simulink model "quad_control_elev8_sAttit"  (Simulink 8.7)
settings: Solver=VariableStepAuto  StartTime=0.0  StopTime=200  FixedStep=0.01  MaxStep=0.1  RelTol=1e-3
InitFcn:
  | ganho=50;
  | z1=0.005;
  | z2=0.001;
  | P_X = (z1+z2)*ganho;      I_X = z1*z2*ganho;     D_X  = ganho;
  | P_Y = (z1+z2)*ganho;      I_Y = z1*z2*ganho;      D_Y  = ganho;
  | P_Z = 32;       I_Z = 3;          D_Z = 15;
  | % --------------------------
  | 
  | global clientID;
  | clientID=-1;
undefined symbols (not defined in the file or in its folder): Angular, Linear, sigbuilder_block
libraries: dspsigops x7, robotlib x7, simulink_extras x3, aerolibutil x1, aerolibtransform2 x1
settings Model: Creator=kleber  LastModifiedBy=kleber
settings DataIOCC: LimitDataPoints=off
settings DebuggingCC: UnderspecifiedInitializationDetection=Simplified  MergeDetectMultiDrivingBlocksExec=error  SolverPrmCheckMsg=warning
settings ConfigComp: CovSFcnEnable=off

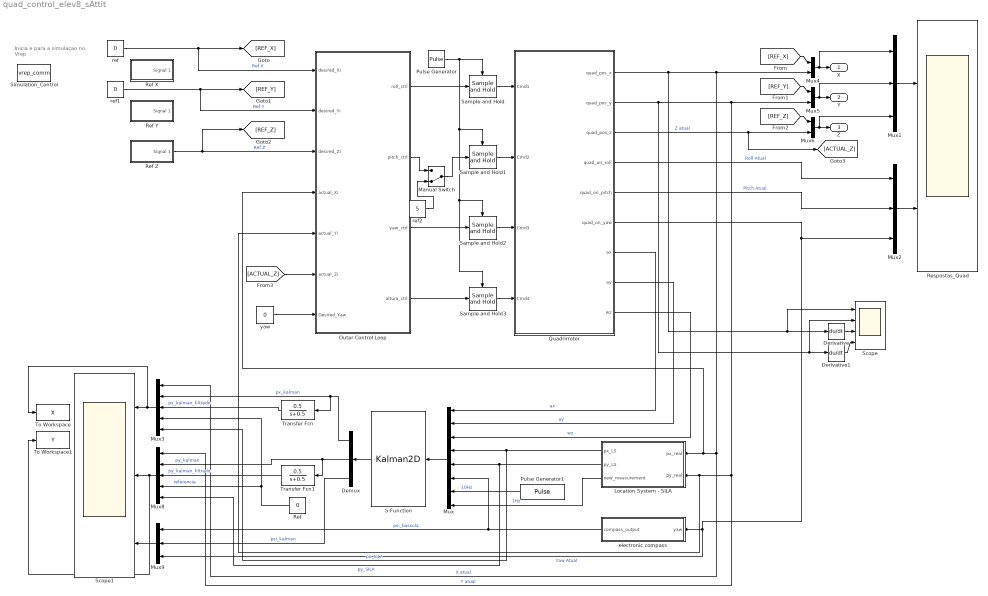
== system quad_control_elev8_sAttit ==
  note: Inicia e para a simulaçao no Vrep
  Demux : Demux  Outputs=3
  Derivative : Derivative
  Derivative1 : Derivative
  Location System - SILA : Subsystem
  Manual Switch : ManualSwitch  CurrentSetting=0
  Mux : Mux  Inputs=8
  Mux1 : Mux  Inputs=3
  Mux2 : Mux  Inputs=3
  Mux3 : Mux  Inputs=5
  Mux4 : Mux  Inputs=2
  Mux5 : Mux  Inputs=2
  Mux6 : Mux  Inputs=2
  Mux8 : Mux  Inputs=5
  Mux9 : Mux  Inputs=3
  Outer Control Loop : Subsystem
  Pulse Generator : DiscretePulseGenerator  PulseType=Time based  Period=0.1  PulseWidth=20  PhaseDelay=0.02
  Pulse Generator1 : DiscretePulseGenerator  PulseType=Time based  Period=0.1  PulseWidth=20
  Quadrirrotor : Subsystem
  Ref : Constant  Value=0
  Ref X : Subsystem  Tag=STV Subsys  LoadFcn=sigbuilder_block('load');  StartFcn=sigbuilder_block('start');  StopFcn=sigbuilder_block('stop');  ClipboardFcn=sigbuilder_block('clipboard');  mask(Sigbuilder block){}
      mask help: Sigbuilder GUI
      mask init:
      | if ~strcmp(get_param(bdroot(gcbh),'SimulationStatus'),'stopped') tuvar = sigbuilder_block('maskInit'); end
      settings: CopyFcn=sigbuilder_block('copy');  DeleteFcn=sigbuilder_block('delete');  ModelCloseFcn=sigbuilder_block('modelClose');  PreSaveFcn=sigbuilder_block('preSave');  PauseFcn=sigbuilder_block('pause')  ContinueFcn=sigbuilder_block('continue')  NameChangeFcn=sigbuilder_block('namechange');  OpenFcn=sigbuilder_block('open',[1024.5 -192 960 708.75 ]);  CloseFcn=sigbuilder_block('close');
      mask Display: plot(0,0,100,100,[10,10,40,40,10],[80,20,20,80,80],[40,10],[50,50], [40,27,10],[65,72,56],[40,25,25,10],[28,28,43,43]);
  Ref Y : Subsystem  Tag=STV Subsys  LoadFcn=sigbuilder_block('load');  StartFcn=sigbuilder_block('start');  StopFcn=sigbuilder_block('stop');  ClipboardFcn=sigbuilder_block('clipboard');  mask(Sigbuilder block){}
      mask help: Sigbuilder GUI
      mask init:
      | if ~strcmp(get_param(bdroot(gcbh),'SimulationStatus'),'stopped') tuvar = sigbuilder_block('maskInit'); end
      settings: CopyFcn=sigbuilder_block('copy');  DeleteFcn=sigbuilder_block('delete');  ModelCloseFcn=sigbuilder_block('modelClose');  PreSaveFcn=sigbuilder_block('preSave');  PauseFcn=sigbuilder_block('pause')  ContinueFcn=sigbuilder_block('continue')  NameChangeFcn=sigbuilder_block('namechange');  OpenFcn=sigbuilder_block('open',[39.75 0 984.75 516.75 ]);  CloseFcn=sigbuilder_block('close');
      mask Display: plot(0,0,100,100,[10,10,40,40,10],[80,20,20,80,80],[40,10],[50,50], [40,27,10],[65,72,56],[40,25,25,10],[28,28,43,43]);
  Ref Z : Subsystem  Tag=STV Subsys  LoadFcn=sigbuilder_block('load');  StartFcn=sigbuilder_block('start');  StopFcn=sigbuilder_block('stop');  ClipboardFcn=sigbuilder_block('clipboard');  mask(Sigbuilder block){}
      mask help: Sigbuilder GUI
      mask init:
      | if ~strcmp(get_param(bdroot(gcbh),'SimulationStatus'),'stopped') tuvar = sigbuilder_block('maskInit'); end
      settings: CopyFcn=sigbuilder_block('copy');  DeleteFcn=sigbuilder_block('delete');  ModelCloseFcn=sigbuilder_block('modelClose');  PreSaveFcn=sigbuilder_block('preSave');  PauseFcn=sigbuilder_block('pause')  ContinueFcn=sigbuilder_block('continue')  NameChangeFcn=sigbuilder_block('namechange');  OpenFcn=sigbuilder_block('open',[43.5 0 981 277.5 ]);  CloseFcn=sigbuilder_block('close');
      mask Display: plot(0,0,100,100,[10,10,40,40,10],[80,20,20,80,80],[40,10],[50,50], [40,27,10],[65,72,56],[40,25,25,10],[28,28,43,43]);
  Respostas_Quad : Scope  NumInputPorts=2
  S-Function : S-Function  FunctionName=Kalman2D  SFunctionDeploymentMode=off  EnableBusSupport=off
  Sample and Hold{,1..3} (4 alike) : dspsigops/Sample and Hold  trig=Rising edge  initCond=0  latchinput=off
  Scope : Scope  NumInputPorts=4
  Scope1 : Scope  NumInputPorts=3
  Simulation_Control : S-Function  FunctionName=vrep_comm  SFunctionDeploymentMode=off  EnableBusSupport=off
  To Workspace : ToWorkspace  VariableName=X  SaveFormat=Timeseries  SampleTime=-1
  To Workspace1 : ToWorkspace  VariableName=Y  SaveFormat=Timeseries  SampleTime=-1
  Transfer Fcn : TransferFcn  Numerator=[0.5]  Denominator=[1 0.5]
  Transfer Fcn1 : TransferFcn  Numerator=[0.5]  Denominator=[1 0.5]
  electronic compass : Subsystem
  ref : Constant  Value=0
  ref1 : Constant  Value=0
  ref2 : Constant  Value=5
  yaw : Constant  Value=0
  X : Outport
  Y : Outport  Port=2
  Z : Outport  Port=3
  wires:
  Mux1/1 -> Respostas_Quad/1
  Mux2/1 -> Respostas_Quad/2
  Quadrirrotor/5(quad_ori_pitch) -> Mux2/2  "Pitch Atual"
  Quadrirrotor/4(quad_ori_roll) -> Mux2/1  "Roll Atual"
  Quadrirrotor/3(quad_pos_z) -> Mux6/2, [ACTUAL_Z]  "Z atual"
  Quadrirrotor/6(quad_ori_yaw) -> Mux9/3, electronic compass/1(yaw), Mux2/3  "Yaw Atual"
  Pulse Generator/1 -> Sample and Hold2/Trigger, Sample and Hold3/Trigger, Sample and Hold1/Trigger, Sample and Hold/Trigger
  Outer Control Loop/4(altura_ctrl) -> Sample and Hold3/1
  Mux4/1 -> X/1, Mux1/1
  Mux5/1 -> Mux1/2, Y/1
  Mux6/1 -> Mux1/3, Z/1
  Outer Control Loop/3(yaw_ctrl) -> Sample and Hold2/1
  Manual Switch/1 -> Sample and Hold1/1
  Outer Control Loop/1(roll_ctrl) -> Sample and Hold/1
  yaw/1 -> Outer Control Loop/7(Desired_Yaw)
  Sample and Hold3/1 -> Quadrirrotor/4(Cmd4)
  Ref Z/1(Signal 1) -> [REF_Z], Outer Control Loop/3(desired_Zi)  "Ref Z"
  Sample and Hold2/1 -> Quadrirrotor/3(Cmd3)
  Mux/1 -> S-Function/1
  Quadrirrotor/7(ax) -> Mux/1  "ax"
  Quadrirrotor/8(ay) -> Mux/2  "ay"
  Quadrirrotor/9(wz) -> Mux/3  "wz"
  Location System - SILA/1(px_LS) -> Mux/4, Mux3/5  "px_SILA"
  Location System - SILA/2(py_LS) -> Mux8/5, Mux/5  "py_SILA"
  [REF_X] -> Mux4/1
  [REF_Y] -> Mux5/1
  [REF_Z] -> Mux6/1
  [ACTUAL_Z] -> Outer Control Loop/6(actual_Zi)
  electronic compass/1(compass_output) -> Mux/6, Mux9/1  "psi_bussola"
  Location System - SILA/3(new_measurement) -> Mux/8  "1Hz"
  S-Function/1 -> Demux/1
  Quadrirrotor/2(quad_pos_y) -> Scope/2, Derivative1/1, Mux5/2, Outer Control Loop/5(actual_Yi), Location System - SILA/2(py_real), Mux8/1  "Y atual"
  Quadrirrotor/1(quad_pos_x) -> Scope/1, Derivative/1, Mux4/2, Outer Control Loop/4(actual_Xi), Location System - SILA/1(px_real), Mux3/1  "X atual"
  Demux/1 -> Transfer Fcn/1, Mux3/2  "px_kalman"
  Mux8/1 -> To Workspace1/1, Scope1/2
  Demux/2 -> Transfer Fcn1/1, Mux8/2  "py_kalman"
  Mux9/1 -> Scope1/3
  Demux/3 -> Mux9/2  "psi_kalman"
  Sample and Hold/1 -> Quadrirrotor/1(Cmd1)
  Transfer Fcn1/1 -> Mux8/3  "py_kalman_filtrado"
  Transfer Fcn/1 -> Mux3/3  "px_kalman_filtrado"
  Sample and Hold1/1 -> Quadrirrotor/2(Cmd2)
  Ref/1 -> Mux3/4, Mux8/4  "referencia"
  Pulse Generator1/1 -> Mux/7  "10Hz"
  ref/1 -> Outer Control Loop/1(desired_Xi), [REF_X]  "Ref X"
  ref1/1 -> Outer Control Loop/2(desired_Yi), [REF_Y]  "Ref Y"
  Mux3/1 -> To Workspace/1, Scope1/1
  Outer Control Loop/2(pitch_ctrl) -> Manual Switch/1
  ref2/1 -> Manual Switch/2
  Derivative/1 -> Scope/3
  Derivative1/1 -> Scope/4

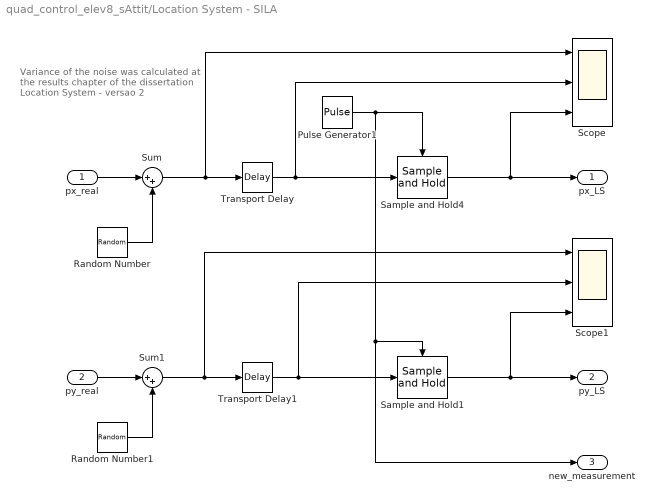
== system quad_control_elev8_sAttit/Location System - SILA ==
  note: Variance of the noise was calculated
      | at the results chapter of the dissertation
      | Location System - versao 2
  px_real : Inport
  py_real : Inport  Port=2
  Pulse Generator1 : DiscretePulseGenerator  PulseType=Time based  Period=1  PulseWidth=10
  Random Number : RandomNumber  Variance=0.0010  SampleTime=1
  Random Number1 : RandomNumber  Variance=0.0012  SampleTime=1
  Sample and Hold1 : dspsigops/Sample and Hold  trig=Rising edge  initCond=0  latchinput=off
  Sample and Hold4 : dspsigops/Sample and Hold  trig=Rising edge  initCond=0  latchinput=off
  Scope : Scope  NumInputPorts=3
  Scope1 : Scope  NumInputPorts=3
  Sum : Sum  Inputs=|++
  Sum1 : Sum  Inputs=|++
  Transport Delay : TransportDelay  DelayTime=0.5
  Transport Delay1 : TransportDelay  DelayTime=0.5
  px_LS : Outport
  py_LS : Outport  Port=2
  new_measurement : Outport  Port=3
  wires:
  Sample and Hold4/1 -> px_LS/1, Scope/3
  Sum/1 -> Transport Delay/1, Scope/1
  Transport Delay/1 -> Sample and Hold4/1, Scope/2
  Sample and Hold1/1 -> py_LS/1, Scope1/3
  Transport Delay1/1 -> Sample and Hold1/1, Scope1/2
  Pulse Generator1/1 -> Sample and Hold4/Trigger, new_measurement/1, Sample and Hold1/Trigger
  px_real/1 -> Sum/1
  Sum1/1 -> Scope1/1, Transport Delay1/1
  py_real/1 -> Sum1/1
  Random Number1/1 -> Sum1/2
  Random Number/1 -> Sum/2

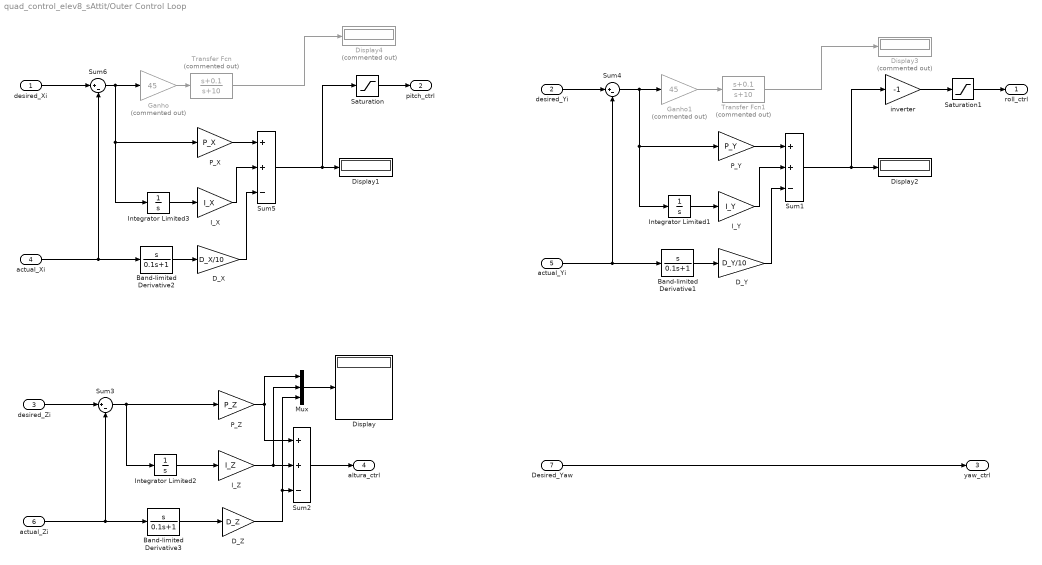
== system quad_control_elev8_sAttit/Outer Control Loop ==
  desired_Xi : Inport
  desired_Yi : Inport  Port=2
  desired_Zi : Inport  Port=3
  actual_Xi : Inport  Port=4
  actual_Yi : Inport  Port=5
  actual_Zi : Inport  Port=6
  Desired_Yaw : Inport  Port=7
  Band-limited Derivative1 : TransferFcn  Numerator=[1 0]  Denominator=[0.1 1]
  Band-limited Derivative2 : TransferFcn  Numerator=[1 0]  Denominator=[0.1 1]
  Band-limited Derivative3 : TransferFcn  Numerator=[1 0]  Denominator=[0.1 1]
  D_X : Gain  Gain=D_X/10
  D_Y : Gain  Gain=D_Y/10
  D_Z : Gain  Gain=D_Z
  Display : Display
  Display1 : Display
  Display2 : Display
  Display3 : Display  Commented=on
  Display4 : Display  Commented=on
  Ganho : Gain  Commented=on  Gain=45
  Ganho1 : Gain  Commented=on  Gain=45
  I_X : Gain  Gain=I_X
  I_Y : Gain  Gain=I_Y
  I_Z : Gain  Gain=I_Z
  Integrator Limited1 : Integrator  LimitOutput=on  UpperSaturationLimit=0.5  LowerSaturationLimit=-0.5
  Integrator Limited2 : Integrator  InitialCondition=1  LimitOutput=on  UpperSaturationLimit=10  LowerSaturationLimit=0
  Integrator Limited3 : Integrator  LimitOutput=on  UpperSaturationLimit=0.5  LowerSaturationLimit=-0.5
  Mux : Mux  Inputs=3
  P_X : Gain  Gain=P_X
  P_Y : Gain  Gain=P_Y
  P_Z : Gain  Gain=P_Z
  Saturation : Saturate  UpperLimit=2  LowerLimit=-2
  Saturation1 : Saturate  UpperLimit=2  LowerLimit=-2
  Sum1 : Sum  Inputs=++-
  Sum2 : Sum  Inputs=++-
  Sum3 : Sum  Inputs=|+-
  Sum4 : Sum  Inputs=|+-
  Sum5 : Sum  Inputs=++-
  Sum6 : Sum  Inputs=|+-
  Transfer Fcn : TransferFcn  Commented=on  Numerator=[1 0.1]  Denominator=[1 10]
  Transfer Fcn1 : TransferFcn  Commented=on  Numerator=[1 0.1]  Denominator=[1 10]
  inverter : Gain  Gain=-1
  roll_ctrl : Outport
  pitch_ctrl : Outport  Port=2
  yaw_ctrl : Outport  Port=3
  altura_ctrl : Outport  Port=4
  wires:
  Sum2/1 -> altura_ctrl/1
  Desired_Yaw/1 -> yaw_ctrl/1
  Saturation/1 -> pitch_ctrl/1
  inverter/1 -> Saturation1/1
  Saturation1/1 -> roll_ctrl/1
  Mux/1 -> Display/1
  Sum3/1 -> Integrator Limited2/1, P_Z/1
  P_Z/1 -> Sum2/1, Mux/1
  D_Z/1 -> Mux/3, Sum2/3
  Band-limited Derivative3/1 -> D_Z/1
  I_Z/1 -> Mux/2, Sum2/2
  Integrator Limited3/1 -> I_X/1
  P_X/1 -> Sum5/1
  D_X/1 -> Sum5/3
  actual_Xi/1 -> Band-limited Derivative2/1, Sum6/2
  desired_Xi/1 -> Sum6/1
  I_X/1 -> Sum5/2
  Integrator Limited2/1 -> I_Z/1
  Integrator Limited1/1 -> I_Y/1
  P_Y/1 -> Sum1/1
  D_Y/1 -> Sum1/3
  actual_Yi/1 -> Band-limited Derivative1/1, Sum4/2
  desired_Yi/1 -> Sum4/1
  I_Y/1 -> Sum1/2
  actual_Zi/1 -> Band-limited Derivative3/1, Sum3/2
  desired_Zi/1 -> Sum3/1
  Sum5/1 -> Saturation/1, Display1/1
  Sum6/1 -> Integrator Limited3/1, P_X/1, Ganho/1
  Ganho/1 -> Transfer Fcn/1
  Ganho1/1 -> Transfer Fcn1/1
  Sum4/1 -> Integrator Limited1/1, P_Y/1, Ganho1/1
  Sum1/1 -> inverter/1, Display2/1
  Band-limited Derivative2/1 -> D_X/1
  Band-limited Derivative1/1 -> D_Y/1
  Transfer Fcn/1 -> Display4/1
  Transfer Fcn1/1 -> Display3/1

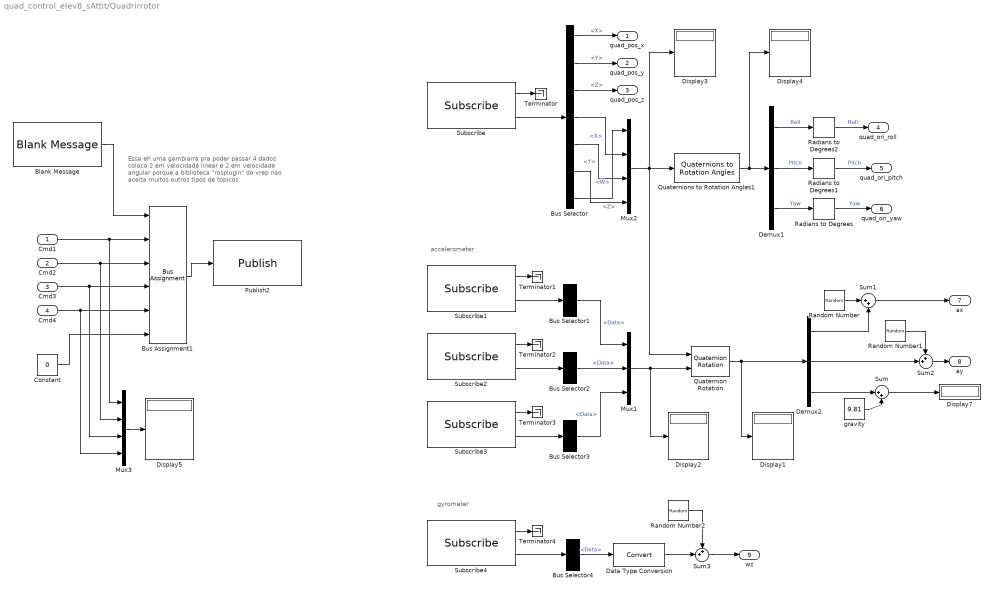
== system quad_control_elev8_sAttit/Quadrirrotor ==
  note: accelerometer
  note: Essa eh uma gambiarra pra poder passar 4 dados coloco 2 em velocidade linear e 2 em velocidade angular porque a biblioteca "rosplugin" do vrep nao aceita muitos outros tipos de topicos
  note: gyrometer
  Cmd1 : Inport
  Cmd2 : Inport  Port=2
  Cmd3 : Inport  Port=3
  Cmd4 : Inport  Port=4
  Blank Message : robotlib/Blank Message  SourceLibraryInfo=This block requires Robotics System Toolbox  messageType=geometry_msgs/Twist  SampleTime=inf
  Bus Assignment1 : BusAssignment  DialogController=Simulink.DDGSource_BusAssignment  AssignedSignals=Linear.X,Linear.Y,Angular.X,Angular.Y,Angular.Z
  Bus Selector : BusSelector  OutputSignals=Pose.Position.X,Pose.Position.Y,Pose.Position.Z,Pose.Orientation.X,Pose.Orientation.Y,Pose.Orientation.Z,Pose.Orientation.W
  Bus Selector{1..4} (4 alike) : BusSelector  OutputSignals=Data
  Constant : Constant  Value=0
  Data Type Conversion : DataTypeConversion
  Demux1 : Demux  Outputs=3
  Demux2 : Demux  Outputs=3
  Display{1..5,7} (6 alike) : Display
  Mux1 : Mux  Inputs=3
  Mux2 : Mux
  Mux3 : Mux
  Publish2 : robotlib/Publish  SourceLibraryInfo=This block requires Robotics System Toolbox  topicSource=Select from ROS network  topic=/control_signals  messageType=geometry_msgs/Twist  messageQueueLength=105
  Quaternion Rotation : aerolibutil/Quaternion Rotation
  Quaternions to Rotation Angles1 : aerolibtransform2/Quaternions to Rotation Angles  rotationOrder=XYZ
  Radians to Degrees : simulink_extras/Transformations/Radians to Degrees
  Radians to Degrees1 : simulink_extras/Transformations/Radians to Degrees
  Radians to Degrees2 : simulink_extras/Transformations/Radians to Degrees
  Random Number : RandomNumber  Variance=0.0023  SampleTime=1
  Random Number1 : RandomNumber  Variance=0.0023  SampleTime=1
  Random Number2 : RandomNumber  Variance=0.000049  SampleTime=1
  Subscribe : robotlib/Subscribe  SourceLibraryInfo=This block requires Robotics System Toolbox  topicSource=Select from ROS network  topic=/quad_pos_ang  messageType=geometry_msgs/PoseStamped  sampleTime=-1  messageQueueLength=51
  Subscribe1 : robotlib/Subscribe  SourceLibraryInfo=This block requires Robotics System Toolbox  topicSource=Select from ROS network  topic=/vrep/quad_aX  messageType=std_msgs/Float32  sampleTime=-1  messageQueueLength=51
  Subscribe2 : robotlib/Subscribe  SourceLibraryInfo=This block requires Robotics System Toolbox  topicSource=Select from ROS network  topic=/vrep/quad_aY  messageType=std_msgs/Float32  sampleTime=-1  messageQueueLength=51
  Subscribe3 : robotlib/Subscribe  SourceLibraryInfo=This block requires Robotics System Toolbox  topicSource=Select from ROS network  topic=/vrep/quad_aZ  messageType=std_msgs/Float32  sampleTime=-1  messageQueueLength=51
  Subscribe4 : robotlib/Subscribe  SourceLibraryInfo=This block requires Robotics System Toolbox  topicSource=Select from ROS network  topic=/vrep/quad_wZ  messageType=std_msgs/Float32  sampleTime=-1  messageQueueLength=51
  Sum : Sum  Inputs=|++
  Sum1 : Sum  Inputs=|++
  Sum2 : Sum  Inputs=++|
  Sum3 : Sum  Inputs=++|
  Terminator{,1..4} (5 alike) : Terminator
  gravity : Constant  Value=9.81
  quad_pos_x : Outport
  quad_pos_y : Outport  Port=2
  quad_pos_z : Outport  Port=3
  quad_ori_roll : Outport  Port=4
  quad_ori_pitch : Outport  Port=5
  quad_ori_yaw : Outport  Port=6
  ax : Outport  Port=7
  ay : Outport  Port=8
  wz : Outport  Port=9
  wires:
  Cmd1/1 -> Bus Assignment1/2, Mux3/1
  Bus Selector/1 -> quad_pos_x/1  "<X>"
  Bus Selector/2 -> quad_pos_y/1  "<Y>"
  Bus Selector/3 -> quad_pos_z/1  "<Z>"
  Radians to Degrees2/1 -> quad_ori_roll/1  "Roll"
  Radians to Degrees1/1 -> quad_ori_pitch/1  "Pitch"
  Radians to Degrees/1 -> quad_ori_yaw/1  "Yaw"
  Demux1/3 -> Radians to Degrees/1  "Yaw"
  Demux1/2 -> Radians to Degrees1/1  "Pitch"
  Demux1/1 -> Radians to Degrees2/1  "Roll"
  Bus Assignment1/1 -> Publish2/1
  Blank Message/1 -> Bus Assignment1/1
  Subscribe/2 -> Bus Selector/1
  Subscribe/1 -> Terminator/1
  Bus Selector/5 -> Mux2/3  "<Y>"
  Bus Selector/6 -> Mux2/4  "<Z>"
  Bus Selector/7 -> Mux2/1  "<W>"
  Mux2/1 -> Display3/1, Quaternions to Rotation Angles1/1, Quaternion Rotation/1
  Bus Selector/4 -> Mux2/2  "<X>"
  Cmd3/1 -> Bus Assignment1/4, Mux3/3
  Cmd4/1 -> Bus Assignment1/5, Mux3/4
  Quaternions to Rotation Angles1/1 -> Display4/1, Demux1/1
  Mux3/1 -> Display5/1
  Cmd2/1 -> Bus Assignment1/3, Mux3/2
  Constant/1 -> Bus Assignment1/6
  Subscribe1/1 -> Terminator1/1
  Subscribe2/1 -> Terminator2/1
  Subscribe3/1 -> Terminator3/1
  Quaternion Rotation/1 -> Demux2/1, Display1/1
  Mux1/1 -> Display2/1, Quaternion Rotation/2
  Subscribe1/2 -> Bus Selector1/1
  Bus Selector1/1 -> Mux1/1  "<Data>"
  Subscribe2/2 -> Bus Selector2/1
  Bus Selector2/1 -> Mux1/2  "<Data>"
  Subscribe3/2 -> Bus Selector3/1
  Bus Selector3/1 -> Mux1/3  "<Data>"
  Demux2/3 -> Sum/1
  Sum/1 -> Display7/1
  gravity/1 -> Sum/2
  Subscribe4/1 -> Terminator4/1
  Subscribe4/2 -> Bus Selector4/1
  Bus Selector4/1 -> Data Type Conversion/1  "<Data>"
  Demux2/1 -> Sum1/2
  Sum2/1 -> ay/1
  Demux2/2 -> Sum2/2
  Sum1/1 -> ax/1
  Data Type Conversion/1 -> Sum3/2
  Random Number2/1 -> Sum3/1
  Sum3/1 -> wz/1
  Random Number/1 -> Sum1/1
  Random Number1/1 -> Sum2/1

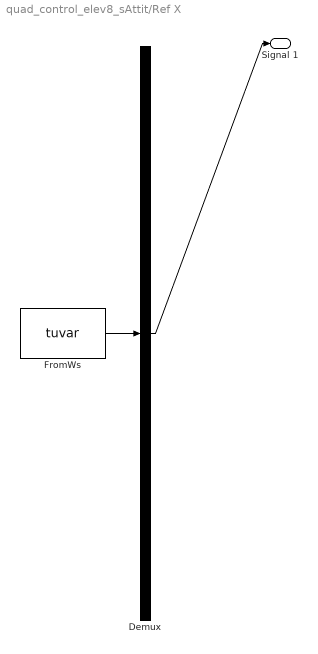
== system quad_control_elev8_sAttit/Ref X ==
  Demux : Demux  Tag=STV Demux  Outputs=1
  FromWs : FromWorkspace  Tag=STV FromWs  VariableName=tuvar  SampleTime=0  SigBuilderData=DataTag0  VnvData=DataTag1
      SigBuilderData=|
      | common.afterFinalStr = 'Extrapolate'
      | common.sampleTime = 0
      | dataSet.timeRange = [0 180]
      | dataSet.name = 'Group 1'
      | sbobj.Name = 'Signal Builder'
      | sbobj.Groups.Name = 'Group 1'
      | sbobj.Groups.Signals.Name = 'Signal 1'
      | sbobj.Groups.Signals.XData = [0 60 90 120 150 160 180]
      | sbobj.Groups.Signals.YData = [0 0 1 1 0 0 0]
      | sbobj.Groups.TimeRange = [0 180]
  Signal 1 : Outport  Tag=STV Outport
  wires:
  FromWs/1 -> Demux/1
  Demux/1 -> Signal 1/1

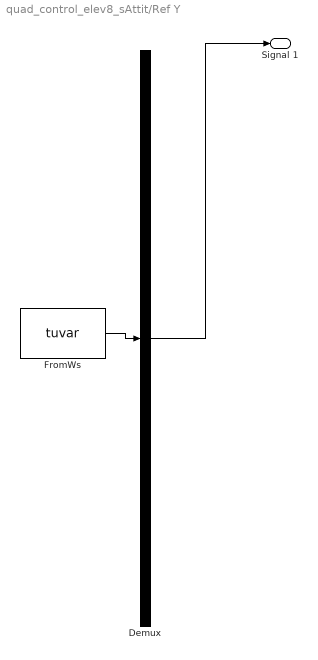
== system quad_control_elev8_sAttit/Ref Y ==
  Demux : Demux  Tag=STV Demux  Outputs=1
  FromWs : FromWorkspace  Tag=STV FromWs  VariableName=tuvar  SampleTime=0  SigBuilderData=DataTag2  VnvData=DataTag3
      SigBuilderData=|
      | common.afterFinalStr = 'Extrapolate'
      | common.sampleTime = 0
      | dataSet.timeRange = [0 180]
      | dataSet.name = 'Group 1'
      | sbobj.Name = 'Signal Builder'
      | sbobj.Groups.Name = 'Group 1'
      | sbobj.Groups.Signals.Name = 'Signal 1'
      | sbobj.Groups.Signals.XData = [0 30 60 120 150 180]
      | sbobj.Groups.Signals.YData = [0 0 1 1 0 0]
      | sbobj.Groups.TimeRange = [0 180]
  Signal 1 : Outport  Tag=STV Outport
  wires:
  Demux/1 -> Signal 1/1
  FromWs/1 -> Demux/1

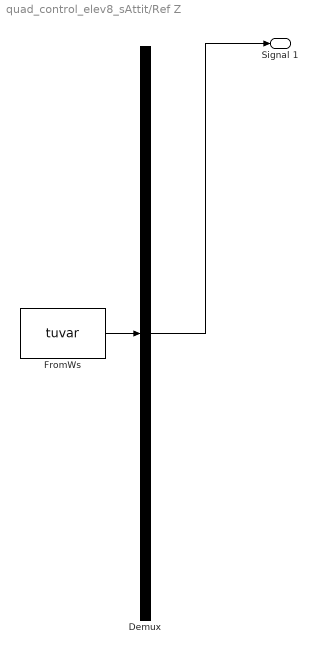
== system quad_control_elev8_sAttit/Ref Z ==
  Demux : Demux  Tag=STV Demux  Outputs=1
  FromWs : FromWorkspace  Tag=STV FromWs  VariableName=tuvar  SampleTime=0  SigBuilderData=DataTag4  VnvData=DataTag5
      SigBuilderData=|
      | common.afterFinalStr = 'Extrapolate'
      | common.sampleTime = 0
      | dataSet.timeRange = [0 180]
      | dataSet.name = 'Group 1'
      | sbobj.Name = 'Signal Builder'
      | sbobj.Groups.Name = 'Group 1'
      | sbobj.Groups.Signals.Name = 'Signal 1'
      | sbobj.Groups.Signals.XData = [0 10 10 180]
      | sbobj.Groups.Signals.YData = [0.1 0.1 0.5 0.5]
      | sbobj.Groups.TimeRange = [0 180]
  Signal 1 : Outport  Tag=STV Outport
  wires:
  Demux/1 -> Signal 1/1
  FromWs/1 -> Demux/1

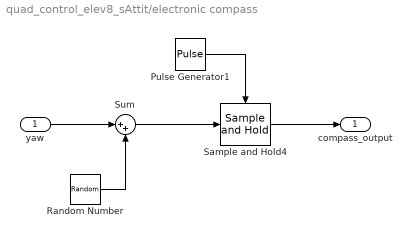
== system quad_control_elev8_sAttit/electronic compass ==
  yaw : Inport
  Pulse Generator1 : DiscretePulseGenerator  PulseType=Time based  Period=1  PulseWidth=10
  Random Number : RandomNumber  SampleTime=1
  Sample and Hold4 : dspsigops/Sample and Hold  trig=Rising edge  initCond=0  latchinput=off
  Sum : Sum  Inputs=|++
  compass_output : Outport
  wires:
  yaw/1 -> Sum/1
  Random Number/1 -> Sum/2
  Pulse Generator1/1 -> Sample and Hold4/Trigger
  Sample and Hold4/1 -> compass_output/1
  Sum/1 -> Sample and Hold4/1
